simulink model "IEEE_30_Bus_System_with_HVDC"  (R2021a)
settings: Solver=FixedStepDiscrete  StartTime=0.0  StopTime=15  FixedStep=Tss  RelTol=1e-3
InitFcn:
  | Tss=5e-5
  | 
  | Pnom = 20e6
  | Vdc = 40e3
  | 
  | Vbreak_on = Vdc + Vdc*150/800
  | Vbreak_off = Vdc
  | break_status_time = 1.0
  | 
  | Rbrk =  Vdc*Vdc/(1.0*Pnom)
  | 
  | Vg1rms = 33e3*1.0118
  | Lg1 = 20e-6
  | Rg1 = 10e-3
  | f1 = 60.0
  | m_f=27
  | fsw = 10000.0
  | Ilpp = 0.1*Pnom/Vg1rms
  | a = 10.0
  | 
  | ffast = 1.0*fsw
  | Tfast = 1.0/ffast
  | 
  | Rdc = Vdc*Vdc/Pnom
  | 
  | R1 = Vg1rms*Vg1rms / (500*Pnom) / 3.0
  | %L1 = 3.0*1.41*Vg1rms / (2*Vdc) * ((2.0/3.0*Vdc - 1.41*Vg1rms) / (Ilpp*fsw))
  | L1=8e-3
  | %Cf1 = (a+1)/(4*pi*pi*fsw*fsw*Lg1)
  | Cf1=4e-6
  | %C_dc = 100e-10*Pnom
  | C_dc=0.02
  | %R_dump = 1.0/(20.0*pi*f1*Cf1)*10000.0/Pnom
  | R_dump=20
  | 
  | p = -0.135*10.0
  | i = -0.004/2.0
  | 
  | Kp_i = 2*L1*fsw*p / Vdc / 2.0
  | Ki_i = 2*L1*fsw*i / Vdc / 2.0
  | 
  | Tsw = 1/fsw
  | 
  | Vg2rms = 33e3*1.0571
  | Lg2 = 20e-6
  | Rg2 = 10e-3
  | f2 = 60.0
  | fsw2 = 10000.0
  | Il2pp = 0.1*Pnom/Vg2rms
  | a2 = 10.0
  | 
  | R2 = Vg2rms*Vg2rms / (500*Pnom) / 3.0
  | %L2 = 3.0*1.41*Vg2rms / (2*Vdc) * ((2.0/3.0*Vdc - 1.41*Vg2rms) / (Il2pp*fsw2))
  | L2=20e-3
  | %Cf2 = (a2+1)/(4*pi*pi*fsw2*fsw2*Lg2)
  | Cf2=9e-6
  | 
  | %R_dump2 = 1.0/(20.0*pi*f2*Cf2)*10000.0/Pnom
  | R_dump2=20
  | 
  | ... (+10 lines)
undefined symbols (not defined in the file): Angle, DiscIntNeverNeededParam, Magnitude, V_890, Vnom1
libraries: spsThreePhasePISectionLineLib x37, spsThreePhaseVIMeasurementLib x32, spsLoadFlowBusLib x30, spsSeriesRLCBranchLib x27, spsThreePhaseSeriesRLCLoadLib x23, spsVoltageMeasurementLib x17, spsCurrentMeasurementLib x15, spsThreePhaseSourceLib x7, pid_lib x7, spsabctodq0Lib x6, spsFirstOrderFilterLib x4, eeGeneralControl x4
(part 2 of 2)

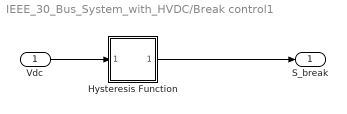
== system IEEE_30_Bus_System_with_HVDC/Break control1 ==
  Vdc : Inport
  Hysteresis Function : Subsystem
  S_break : Outport
  wires:
  Vdc/1 -> Hysteresis Function/1(Input)
  Hysteresis Function/1(Output) -> S_break/1

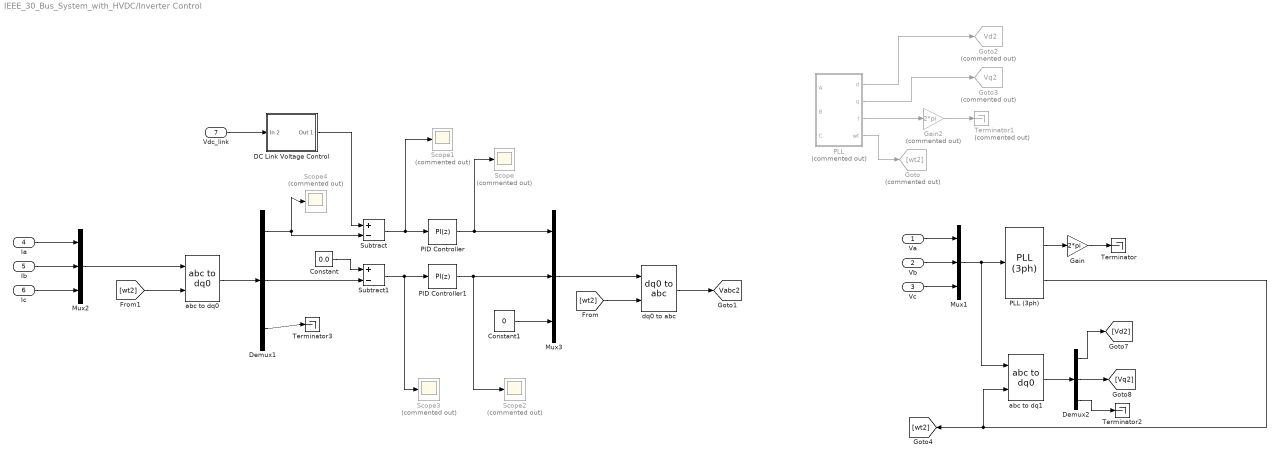
== system IEEE_30_Bus_System_with_HVDC/Inverter Control ==
  Va : Inport
  Vb : Inport  Port=2
  Vc : Inport  Port=3
  Ia : Inport  Port=4
  Ib : Inport  Port=5
  Ic : Inport  Port=6
  Vdc_link : Inport  Port=7
  Constant : Constant  Value=0.0  SampleTime=Tsw2
  Constant1 : Constant  Value=0
  DC Link Voltage Control : Subsystem
  Demux1 : Demux  Outputs=3
  Demux2 : Demux  Outputs=3
  Gain : Gain  Gain=2*pi
  Gain2 : Gain  Commented=on  Gain=2*pi
  Goto : Goto  Commented=on  GotoTag=wt2
  Goto2 : Goto  Commented=on  GotoTag=Vd2  TagVisibility=global
  Goto3 : Goto  Commented=on  GotoTag=Vq2  TagVisibility=global
  Mux1 : Mux  Inputs=3
  Mux2 : Mux  Inputs=3
  Mux3 : Mux  Inputs=3
  PID Controller : pid_lib/PID Controller  Controller=PI  Form=Parallel  TimeDomain=Discrete-time  UseExternalTs=off  SampleTime=-1  IntegratorMethod=Forward Euler  FilterMethod=Forward Euler  ControllerParametersSource=internal  P=Kp_i  I=Ki_i/Tsw2  D=0  UseFilter=on  N=100  TunerSelectOption=Transfer Function Based (PID Tuner App)  InitialConditionSource=internal  InitialConditionForIntegrator=0  InitialConditionForFilter=0  DifferentiatorICPrevScaledInput=0  ExternalReset=none  TrackingMode=off  Kt=1  LimitOutput=on  SatLimitsSource=internal  UpperSaturationLimit=1  LowerSaturationLimit=-1  LinearizeAsGain=on  AntiWindupMode=back-calculation  Kb=Ki_i/Tsw2  POutMin=[]  POutMax=[]  IOutMin=[]  IOutMax=[]  DOutMin=[]  DOutMax=[]  NOutMin=[]  NOutMax=[]  SumOutMin=[]  SumOutMax=[]  SaturationOutMin=[]  SaturationOutMax=[]  PParamMin=[]  PParamMax=[]  IParamMin=[]  IParamMax=[]  DParamMin=[]  DParamMax=[]  NParamMin=[]  NParamMax=[]  KbParamMin=[]  KbParamMax=[]  KtParamMin=[]  KtParamMax=[]  KbOutMin=[]  KbOutMax=[]  KtOutMin=[]  KtOutMax=[]  IntegratorOutMin=[]  IntegratorOutMax=[]  FilterOutMin=[]  FilterOutMax=[]  SumI1OutMin=[]  SumI1OutMax=[]  SumI2OutMin=[]  SumI2OutMax=[]  SumI3OutMin=[]  SumI3OutMax=[]  SumI4OutMin=[]  SumI4OutMax=[]  SumDOutMin=[]  SumDOutMax=[]  DifferentiatorOutMin=[]  DifferentiatorOutMax=[]  FilterDiffOutCoefMin=[]  FilterDiffOutCoefMax=[]  ReciprocalOutMin=[]  ReciprocalOutMax=[]  SumDenOutMin=[]  SumDenOutMax=[]  SumNumOutMin=[]  SumNumOutMax=[]  DivideOutMin=[]  DivideOutMax=[]  UdiffTsProdOutMin=[]  UdiffTsProdOutMax=[]  NTsProdOutMin=[]  NTsProdOutMax=[]  UintegralTsProdOutMin=[]  UintegralTsProdOutMax=[]  UngainTsProdOutMin=[]  UngainTsProdOutMax=[]  IntegratorContinuousStateAttributes=''  IntegratorStateMustResolveToSignalObject=off  IntegratorRTWStateStorageClass=Auto  FilterContinuousStateAttributes=''  FilterStateMustResolveToSignalObject=off  FilterRTWStateStorageClass=Auto  ParallelPVariant=InternalParameters  IdealPVariant=Disabled  IVariant=InternalParameters  DVariant=Disabled  IntegratorVariant=Discrete  SatVariant=Enabled  AWVariant=BackCalculation  PCopyVariant=Disabled  TRVariant=Disabled  FdbkBlocksVariant=Forward  IdealPFdbkVariant=Disabled  SatFdbkVariant=Disabled  DerivativeFilterVariant=Disabled  NVariant=Disabled  NCopyVariant=Disabled_SignalSpec  FilterICVariant=Disabled  IntegratorICVariant=InternalICs  ExternalResetVariant=Disabled  TRSumVariant=Passthrough  SumFdbkVariant=Disabled  SumVariant=Sum_PI  TsampFilterVariant=InternalTs  TsampNgainVariant=Passthrough  TsampIntegralVariant=Passthrough  ExternalSaturationOutDataTypeStr=Inherit: Same as second input
  PID Controller1 : pid_lib/PID Controller  Controller=PI  Form=Parallel  TimeDomain=Discrete-time  UseExternalTs=off  SampleTime=-1  IntegratorMethod=Forward Euler  FilterMethod=Forward Euler  ControllerParametersSource=internal  P=Kp_i  I=Ki_i/Tsw2  D=0  UseFilter=on  N=100  TunerSelectOption=Transfer Function Based (PID Tuner App)  InitialConditionSource=internal  InitialConditionForIntegrator=0  InitialConditionForFilter=0  DifferentiatorICPrevScaledInput=0  ExternalReset=none  TrackingMode=off  Kt=1  LimitOutput=on  SatLimitsSource=internal  UpperSaturationLimit=1  LowerSaturationLimit=-1  LinearizeAsGain=on  AntiWindupMode=back-calculation  Kb=Ki_i/Tsw2  POutMin=[]  POutMax=[]  IOutMin=[]  IOutMax=[]  DOutMin=[]  DOutMax=[]  NOutMin=[]  NOutMax=[]  SumOutMin=[]  SumOutMax=[]  SaturationOutMin=[]  SaturationOutMax=[]  PParamMin=[]  PParamMax=[]  IParamMin=[]  IParamMax=[]  DParamMin=[]  DParamMax=[]  NParamMin=[]  NParamMax=[]  KbParamMin=[]  KbParamMax=[]  KtParamMin=[]  KtParamMax=[]  KbOutMin=[]  KbOutMax=[]  KtOutMin=[]  KtOutMax=[]  IntegratorOutMin=[]  IntegratorOutMax=[]  FilterOutMin=[]  FilterOutMax=[]  SumI1OutMin=[]  SumI1OutMax=[]  SumI2OutMin=[]  SumI2OutMax=[]  SumI3OutMin=[]  SumI3OutMax=[]  SumI4OutMin=[]  SumI4OutMax=[]  SumDOutMin=[]  SumDOutMax=[]  DifferentiatorOutMin=[]  DifferentiatorOutMax=[]  FilterDiffOutCoefMin=[]  FilterDiffOutCoefMax=[]  ReciprocalOutMin=[]  ReciprocalOutMax=[]  SumDenOutMin=[]  SumDenOutMax=[]  SumNumOutMin=[]  SumNumOutMax=[]  DivideOutMin=[]  DivideOutMax=[]  UdiffTsProdOutMin=[]  UdiffTsProdOutMax=[]  NTsProdOutMin=[]  NTsProdOutMax=[]  UintegralTsProdOutMin=[]  UintegralTsProdOutMax=[]  UngainTsProdOutMin=[]  UngainTsProdOutMax=[]  IntegratorContinuousStateAttributes=''  IntegratorStateMustResolveToSignalObject=off  IntegratorRTWStateStorageClass=Auto  FilterContinuousStateAttributes=''  FilterStateMustResolveToSignalObject=off  FilterRTWStateStorageClass=Auto  ParallelPVariant=InternalParameters  IdealPVariant=Disabled  IVariant=InternalParameters  DVariant=Disabled  IntegratorVariant=Discrete  SatVariant=Enabled  AWVariant=BackCalculation  PCopyVariant=Disabled  TRVariant=Disabled  FdbkBlocksVariant=Forward  IdealPFdbkVariant=Disabled  SatFdbkVariant=Disabled  DerivativeFilterVariant=Disabled  NVariant=Disabled  NCopyVariant=Disabled_SignalSpec  FilterICVariant=Disabled  IntegratorICVariant=InternalICs  ExternalResetVariant=Disabled  TRSumVariant=Passthrough  SumFdbkVariant=Disabled  SumVariant=Sum_PI  TsampFilterVariant=InternalTs  TsampNgainVariant=Passthrough  TsampIntegralVariant=Passthrough  ExternalSaturationOutDataTypeStr=Inherit: Same as second input
  PLL : Subsystem  Commented=on
  PLL (3ph) : spsPLL3phLib/PLL (3ph)  Fmin=45  Par_Init=[0, 60]  ParK=[100, 3200, 1]  TcD=1e-4  MaxRateChangeFreq=12  FilterCutOffFreq=25  Ts=Tss  AGC=on
  Scope{,1..4} (5 alike) : Scope  Commented=on
  Subtract : Sum  Inputs=+-
  Subtract1 : Sum  Inputs=+-
  Terminator : Terminator
  Terminator1 : Terminator  Commented=on
  Terminator2 : Terminator
  Terminator3 : Terminator
  abc to dq0 : spsabctodq0Lib/abc to dq0  Alignment=90 degrees behind phase A axis
  abc to dq1 : spsabctodq0Lib/abc to dq0  Alignment=90 degrees behind phase A axis
  dq0 to abc : spsdq0toabcLib/dq0 to abc  Alignment=90 degrees behind phase A axis
  tag scope: Vabc2=global
  wires:
  Ia/1 -> Mux2/1
  Ib/1 -> Mux2/2
  Ic/1 -> Mux2/3
  Mux2/1 -> abc to dq0/1
  abc to dq0/1 -> Demux1/1
  Demux1/2 -> Subtract1/2
  Constant/1 -> Subtract1/1
  Subtract/1 -> Scope1/1, PID Controller/1
  Subtract1/1 -> Scope3/1, PID Controller1/1
  PID Controller/1 -> Scope/1, Mux3/1
  PID Controller1/1 -> Scope2/1, Mux3/2
  Mux3/1 -> dq0 to abc/1
  DC Link Voltage Control/1(Out 1) -> Subtract/1
  PLL/4(wt) -> Goto/1
  PLL/1(d) -> Goto2/1
  PLL/2(q) -> Goto3/1
  Gain2/1 -> Terminator1/1
  PLL/3(f) -> Gain2/1
  Demux2/1 -> [Vd2]
  Gain/1 -> Terminator/1
  Vc/1 -> Mux1/3
  abc to dq1/1 -> Demux2/1
  PLL (3ph)/1 -> Gain/1
  Demux2/2 -> [Vq2]
  Va/1 -> Mux1/1
  Vb/1 -> Mux1/2
  Mux1/1 -> abc to dq1/1, PLL (3ph)/1
  PLL (3ph)/2 -> [wt2], abc to dq1/2
  [wt2] -> dq0 to abc/2
  [wt2] -> abc to dq0/2
  Vdc_link/1 -> DC Link Voltage Control/1(In 2)
  Demux1/1 -> Scope4/1, Subtract/2
  Demux1/3 -> Terminator3/1
  dq0 to abc/1 -> [Vabc2]
  Constant1/1 -> Mux3/3
  Demux2/3 -> Terminator2/1

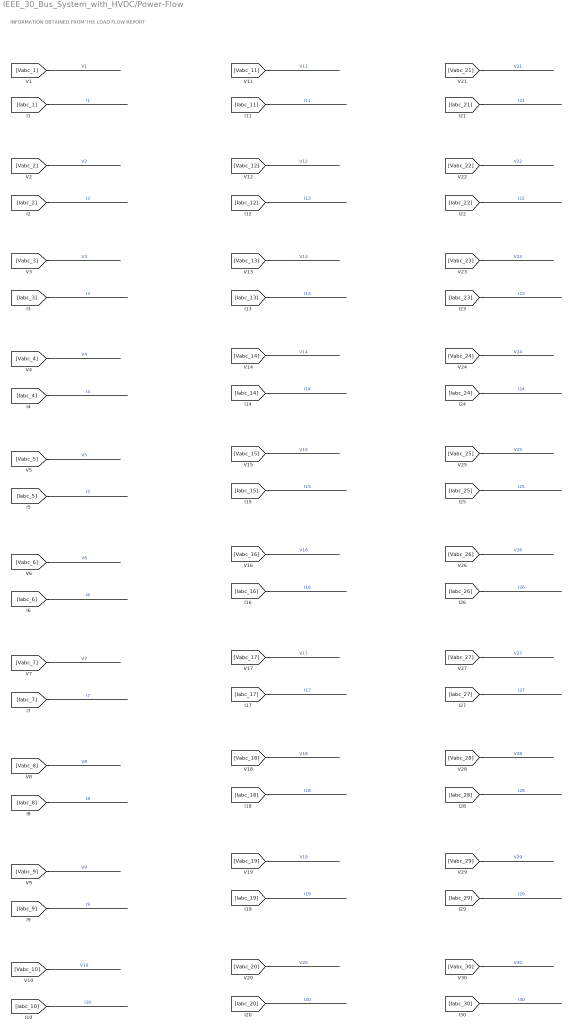
== system IEEE_30_Bus_System_with_HVDC/Power-Flow ==
  note: INFORMATION OBTAINED FROM THE LOAD FLOW REPORT
  wires:
  [Vabc_1] -> ?  "V1"
  [Iabc_1] -> ?  "I1"
  [Vabc_2] -> ?  "V2"
  [Iabc_2] -> ?  "I2"
  [Iabc_3] -> ?  "I3"
  [Vabc_3] -> ?  "V3"
  [Vabc_4] -> ?  "V4"
  [Iabc_4] -> ?  "I4"
  [Vabc_5] -> ?  "V5"
  [Iabc_5] -> ?  "I5"
  [Vabc_6] -> ?  "V6"
  [Iabc_6] -> ?  "I6"
  [Vabc_7] -> ?  "V7"
  [Iabc_7] -> ?  "I7"
  [Vabc_8] -> ?  "V8"
  [Iabc_8] -> ?  "I8"
  [Vabc_9] -> ?  "V9"
  [Iabc_9] -> ?  "I9"
  [Vabc_10] -> ?  "V10"
  [Iabc_10] -> ?  "I10"
  [Iabc_18] -> ?  "I18"
  [Vabc_18] -> ?  "V18"
  [Iabc_13] -> ?  "I13"
  [Vabc_13] -> ?  "V13"
  [Iabc_11] -> ?  "I11"
  [Vabc_16] -> ?  "V16"
  [Iabc_16] -> ?  "I16"
  [Iabc_17] -> ?  "I17"
  [Vabc_17] -> ?  "V17"
  [Vabc_11] -> ?  "V11"
  [Iabc_12] -> ?  "I12"
  [Vabc_20] -> ?  "V20"
  [Iabc_20] -> ?  "I20"
  [Vabc_12] -> ?  "V12"
  [Iabc_19] -> ?  "I19"
  [Iabc_15] -> ?  "I15"
  [Vabc_19] -> ?  "V19"
  [Vabc_15] -> ?  "V15"
  [Vabc_14] -> ?  "V14"
  [Iabc_14] -> ?  "I14"
  [Iabc_26] -> ?  "I26"
  [Vabc_27] -> ?  "V27"
  [Vabc_26] -> ?  "V26"
  [Iabc_21] -> ?  "I21"
  [Vabc_23] -> ?  "V23"
  [Vabc_28] -> ?  "V28"
  [Iabc_27] -> ?  "I27"
  [Iabc_28] -> ?  "I28"
  [Vabc_24] -> ?  "V24"
  [Vabc_25] -> ?  "V25"
  [Iabc_23] -> ?  "I23"
  [Vabc_29] -> ?  "V29"
  [Iabc_24] -> ?  "I24"
  [Iabc_25] -> ?  "I25"
  [Vabc_30] -> ?  "V30"
  [Vabc_22] -> ?  "V22"
  [Iabc_29] -> ?  "I29"
  [Iabc_22] -> ?  "I22"
  [Iabc_30] -> ?  "I30"
  [Vabc_21] -> ?  "V21"

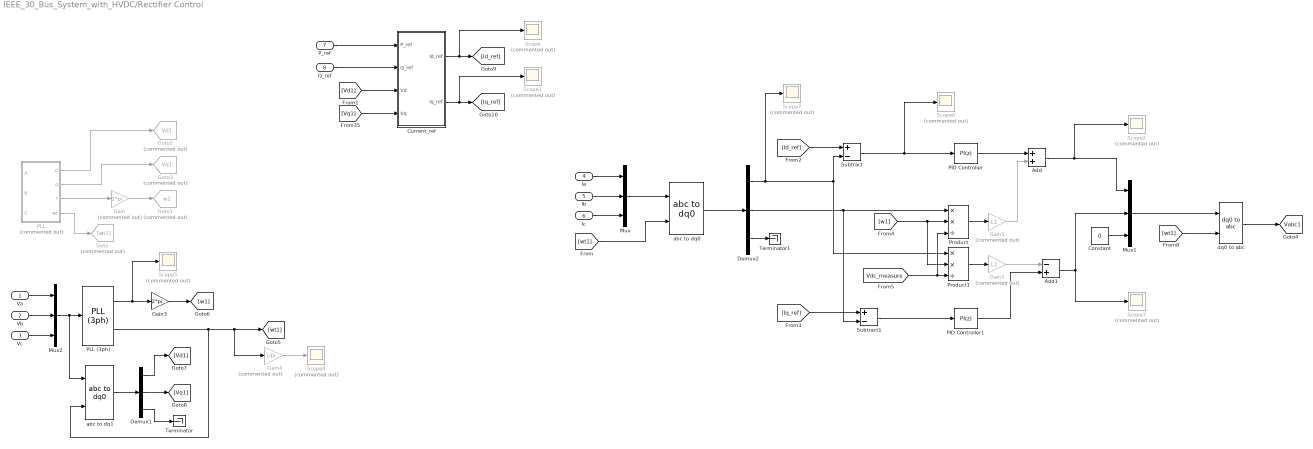
== system IEEE_30_Bus_System_with_HVDC/Rectifier Control ==
  Va : Inport
  Vb : Inport  Port=2
  Vc : Inport  Port=3
  Ia : Inport  Port=4
  Ib : Inport  Port=5
  Ic : Inport  Port=6
  P_ref : Inport  Port=7
  Q_ref : Inport  Port=8
  Add : Sum
  Add1 : Sum  Inputs=-+
  Constant : Constant  Value=0
  Current_ref : Subsystem
  Demux1 : Demux  Outputs=3
  Demux2 : Demux  Outputs=3
  Gain : Gain  Commented=on  Gain=2*pi
  Gain1 : Gain  Commented=on  Gain=L1
  Gain2 : Gain  Commented=on  Gain=L1
  Gain3 : Gain  Gain=2*pi
  Gain4 : Gain  Commented=on  Gain=1/pi
  Goto : Goto  Commented=on  GotoTag=wt1
  Goto1 : Goto  Commented=on  GotoTag=w1  TagVisibility=global
  Goto2 : Goto  Commented=on  GotoTag=Vd1  TagVisibility=global
  Goto3 : Goto  Commented=on  GotoTag=Vq1  TagVisibility=global
  Mux : Mux  Inputs=3
  Mux1 : Mux  Inputs=3
  Mux2 : Mux  Inputs=3
  PID Controller : pid_lib/PID Controller  Controller=PI  Form=Parallel  TimeDomain=Discrete-time  UseExternalTs=off  SampleTime=-1  IntegratorMethod=Forward Euler  FilterMethod=Forward Euler  ControllerParametersSource=internal  P=Kp_i  I=Ki_i/Tsw  D=0  UseFilter=on  N=100  TunerSelectOption=Transfer Function Based (PID Tuner App)  InitialConditionSource=internal  InitialConditionForIntegrator=0  InitialConditionForFilter=0  DifferentiatorICPrevScaledInput=0  ExternalReset=none  TrackingMode=off  Kt=1  LimitOutput=on  SatLimitsSource=internal  UpperSaturationLimit=1  LowerSaturationLimit=-1  LinearizeAsGain=on  AntiWindupMode=back-calculation  Kb=Ki_i/Tsw  POutMin=[]  POutMax=[]  IOutMin=[]  IOutMax=[]  DOutMin=[]  DOutMax=[]  NOutMin=[]  NOutMax=[]  SumOutMin=[]  SumOutMax=[]  SaturationOutMin=[]  SaturationOutMax=[]  PParamMin=[]  PParamMax=[]  IParamMin=[]  IParamMax=[]  DParamMin=[]  DParamMax=[]  NParamMin=[]  NParamMax=[]  KbParamMin=[]  KbParamMax=[]  KtParamMin=[]  KtParamMax=[]  KbOutMin=[]  KbOutMax=[]  KtOutMin=[]  KtOutMax=[]  IntegratorOutMin=[]  IntegratorOutMax=[]  FilterOutMin=[]  FilterOutMax=[]  SumI1OutMin=[]  SumI1OutMax=[]  SumI2OutMin=[]  SumI2OutMax=[]  SumI3OutMin=[]  SumI3OutMax=[]  SumI4OutMin=[]  SumI4OutMax=[]  SumDOutMin=[]  SumDOutMax=[]  DifferentiatorOutMin=[]  DifferentiatorOutMax=[]  FilterDiffOutCoefMin=[]  FilterDiffOutCoefMax=[]  ReciprocalOutMin=[]  ReciprocalOutMax=[]  SumDenOutMin=[]  SumDenOutMax=[]  SumNumOutMin=[]  SumNumOutMax=[]  DivideOutMin=[]  DivideOutMax=[]  UdiffTsProdOutMin=[]  UdiffTsProdOutMax=[]  NTsProdOutMin=[]  NTsProdOutMax=[]  UintegralTsProdOutMin=[]  UintegralTsProdOutMax=[]  UngainTsProdOutMin=[]  UngainTsProdOutMax=[]  IntegratorContinuousStateAttributes=''  IntegratorStateMustResolveToSignalObject=off  IntegratorRTWStateStorageClass=Auto  FilterContinuousStateAttributes=''  FilterStateMustResolveToSignalObject=off  FilterRTWStateStorageClass=Auto  ParallelPVariant=InternalParameters  IdealPVariant=Disabled  IVariant=InternalParameters  DVariant=Disabled  IntegratorVariant=Discrete  SatVariant=Enabled  AWVariant=BackCalculation  PCopyVariant=Disabled  TRVariant=Disabled  FdbkBlocksVariant=Forward  IdealPFdbkVariant=Disabled  SatFdbkVariant=Disabled  DerivativeFilterVariant=Disabled  NVariant=Disabled  NCopyVariant=Disabled_SignalSpec  FilterICVariant=Disabled  IntegratorICVariant=InternalICs  ExternalResetVariant=Disabled  TRSumVariant=Passthrough  SumFdbkVariant=Disabled  SumVariant=Sum_PI  TsampFilterVariant=InternalTs  TsampNgainVariant=Passthrough  TsampIntegralVariant=Passthrough  ExternalSaturationOutDataTypeStr=Inherit: Same as second input
  PID Controller1 : pid_lib/PID Controller  Controller=PI  Form=Parallel  TimeDomain=Discrete-time  UseExternalTs=off  SampleTime=-1  IntegratorMethod=Forward Euler  FilterMethod=Forward Euler  ControllerParametersSource=internal  P=Kp_i  I=Ki_i/Tsw  D=0  UseFilter=on  N=100  TunerSelectOption=Transfer Function Based (PID Tuner App)  InitialConditionSource=internal  InitialConditionForIntegrator=0  InitialConditionForFilter=0  DifferentiatorICPrevScaledInput=0  ExternalReset=none  TrackingMode=off  Kt=1  LimitOutput=on  SatLimitsSource=internal  UpperSaturationLimit=1  LowerSaturationLimit=-1  LinearizeAsGain=on  AntiWindupMode=back-calculation  Kb=Ki_i/Tsw  POutMin=[]  POutMax=[]  IOutMin=[]  IOutMax=[]  DOutMin=[]  DOutMax=[]  NOutMin=[]  NOutMax=[]  SumOutMin=[]  SumOutMax=[]  SaturationOutMin=[]  SaturationOutMax=[]  PParamMin=[]  PParamMax=[]  IParamMin=[]  IParamMax=[]  DParamMin=[]  DParamMax=[]  NParamMin=[]  NParamMax=[]  KbParamMin=[]  KbParamMax=[]  KtParamMin=[]  KtParamMax=[]  KbOutMin=[]  KbOutMax=[]  KtOutMin=[]  KtOutMax=[]  IntegratorOutMin=[]  IntegratorOutMax=[]  FilterOutMin=[]  FilterOutMax=[]  SumI1OutMin=[]  SumI1OutMax=[]  SumI2OutMin=[]  SumI2OutMax=[]  SumI3OutMin=[]  SumI3OutMax=[]  SumI4OutMin=[]  SumI4OutMax=[]  SumDOutMin=[]  SumDOutMax=[]  DifferentiatorOutMin=[]  DifferentiatorOutMax=[]  FilterDiffOutCoefMin=[]  FilterDiffOutCoefMax=[]  ReciprocalOutMin=[]  ReciprocalOutMax=[]  SumDenOutMin=[]  SumDenOutMax=[]  SumNumOutMin=[]  SumNumOutMax=[]  DivideOutMin=[]  DivideOutMax=[]  UdiffTsProdOutMin=[]  UdiffTsProdOutMax=[]  NTsProdOutMin=[]  NTsProdOutMax=[]  UintegralTsProdOutMin=[]  UintegralTsProdOutMax=[]  UngainTsProdOutMin=[]  UngainTsProdOutMax=[]  IntegratorContinuousStateAttributes=''  IntegratorStateMustResolveToSignalObject=off  IntegratorRTWStateStorageClass=Auto  FilterContinuousStateAttributes=''  FilterStateMustResolveToSignalObject=off  FilterRTWStateStorageClass=Auto  ParallelPVariant=InternalParameters  IdealPVariant=Disabled  IVariant=InternalParameters  DVariant=Disabled  IntegratorVariant=Discrete  SatVariant=Enabled  AWVariant=BackCalculation  PCopyVariant=Disabled  TRVariant=Disabled  FdbkBlocksVariant=Forward  IdealPFdbkVariant=Disabled  SatFdbkVariant=Disabled  DerivativeFilterVariant=Disabled  NVariant=Disabled  NCopyVariant=Disabled_SignalSpec  FilterICVariant=Disabled  IntegratorICVariant=InternalICs  ExternalResetVariant=Disabled  TRSumVariant=Passthrough  SumFdbkVariant=Disabled  SumVariant=Sum_PI  TsampFilterVariant=InternalTs  TsampNgainVariant=Passthrough  TsampIntegralVariant=Passthrough  ExternalSaturationOutDataTypeStr=Inherit: Same as second input
  PLL : Subsystem  Commented=on
  PLL (3ph) : spsPLL3phLib/PLL (3ph)  Fmin=45  Par_Init=[0, 60]  ParK=[100, 3200, 1]  TcD=1e-4  MaxRateChangeFreq=12  FilterCutOffFreq=25  Ts=Tss  AGC=on
  Product : Product  Inputs=**/
  Product1 : Product  Inputs=**/
  Scope{,1..7} (8 alike) : Scope  Commented=on
  Subtract : Sum  Inputs=+-
  Subtract1 : Sum  Inputs=+-
  Terminator : Terminator
  Terminator1 : Terminator
  abc to dq0 : spsabctodq0Lib/abc to dq0  Alignment=90 degrees behind phase A axis
  abc to dq1 : spsabctodq0Lib/abc to dq0  Alignment=90 degrees behind phase A axis
  dq0 to abc : spsdq0toabcLib/dq0 to abc  Alignment=90 degrees behind phase A axis
  tag scope: Vabc1=global
  wires:
  PLL/4(wt) -> Goto/1
  PLL/3(f) -> Gain/1
  Gain/1 -> Goto1/1
  PLL/1(d) -> Goto2/1
  PLL/2(q) -> Goto3/1
  [wt1] -> abc to dq0/2
  abc to dq0/1 -> Demux2/1
  Demux2/3 -> Terminator1/1
  Mux/1 -> abc to dq0/1
  Demux2/1 -> Scope7/1, Product1/1, Subtract/2
  Demux2/2 -> Subtract1/2, Product/1
  [w1] -> Product1/2, Product/2
  [Vdc_measure] -> Product/3, Product1/3
  [wt1] -> dq0 to abc/2
  Subtract/1 -> Scope6/1, PID Controller/1
  Subtract1/1 -> PID Controller1/1
  PID Controller1/1 -> Add1/2
  Product/1 -> Gain1/1
  Product1/1 -> Gain2/1
  Gain2/1 -> Add1/1
  dq0 to abc/1 -> [Vabc1]
  Ia/1 -> Mux/1
  Ic/1 -> Mux/3
  Ib/1 -> Mux/2
  Add/1 -> Mux1/1, Scope2/1
  PID Controller/1 -> Add/1
  Gain1/1 -> Add/2
  Demux1/2 -> [Vq1]
  abc to dq1/1 -> Demux1/1
  Mux2/1 -> abc to dq1/1, PLL (3ph)/1
  PLL (3ph)/1 -> Scope5/1, Gain3/1
  Gain3/1 -> [w1]
  Demux1/1 -> [Vd1]
  PLL (3ph)/2 -> abc to dq1/2, Gain4/1, [wt1]
  [Vq1] -> Current_ref/4(Vq)
  [Vd1] -> Current_ref/3(Vd)
  Mux1/1 -> dq0 to abc/1
  Add1/1 -> Mux1/2, Scope3/1
  Constant/1 -> Mux1/3
  P_ref/1 -> Current_ref/1(P_ref)
  Demux1/3 -> Terminator/1
  Va/1 -> Mux2/1
  Vb/1 -> Mux2/2
  Vc/1 -> Mux2/3
  Q_ref/1 -> Current_ref/2(Q_ref)
  Current_ref/1(Id_ref) -> Scope/1, [Id_ref]
  Current_ref/2(Iq_ref) -> Scope1/1, [Iq_ref]
  [Id_ref] -> Subtract/1
  [Iq_ref] -> Subtract1/1
  Gain4/1 -> Scope4/1

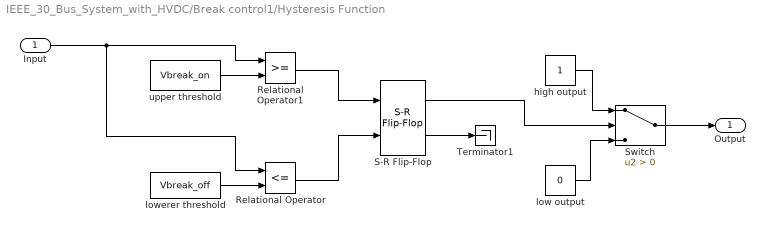
== system IEEE_30_Bus_System_with_HVDC/Break control1/Hysteresis Function ==
  Input : Inport
  Relational Operator : RelationalOperator  Operator=<=  OutDataTypeStr=boolean  RndMeth=Simplest
  Relational Operator1 : RelationalOperator  OutDataTypeStr=boolean  RndMeth=Simplest
  S-R Flip-Flop : simulink_extras/Flip Flops/S-R Flip-Flop  initial_condition=0
  Switch : Switch  Criteria=u2 > Threshold
  Terminator1 : Terminator
  high output : Constant  SampleTime=Tfast
  low output : Constant  Value=0  SampleTime=Tfast
  lowerer threshold : Constant  Value=Vbreak_off  SampleTime=Tfast
  upper threshold : Constant  Value=Vbreak_on  SampleTime=Tfast
  Output : Outport
  wires:
  lowerer threshold/1 -> Relational Operator/2
  upper threshold/1 -> Relational Operator1/2
  Relational Operator1/1 -> S-R Flip-Flop/1
  Relational Operator/1 -> S-R Flip-Flop/2
  S-R Flip-Flop/2 -> Terminator1/1
  S-R Flip-Flop/1 -> Switch/2
  high output/1 -> Switch/1
  low output/1 -> Switch/3
  Input/1 -> Relational Operator1/1, Relational Operator/1
  Switch/1 -> Output/1

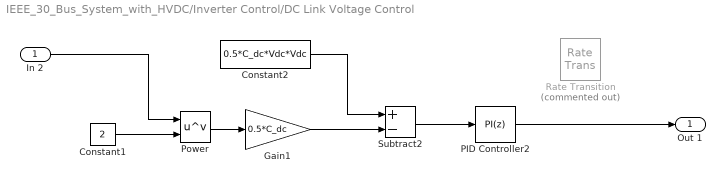
== system IEEE_30_Bus_System_with_HVDC/Inverter Control/DC Link Voltage Control ==
  In 2 : Inport
  Constant1 : Constant  Value=2  SampleTime=Tslow
  Constant2 : Constant  Value=0.5*C_dc*Vdc*Vdc  SampleTime=Tslow
  Gain1 : Gain  Gain=0.5*C_dc
  PID Controller2 : pid_lib/PID Controller  Controller=PI  Form=Parallel  TimeDomain=Discrete-time  UseExternalTs=off  SampleTime=-1  IntegratorMethod=Forward Euler  FilterMethod=Forward Euler  ControllerParametersSource=internal  P=Kp_v  I=Ki_v/Tslow  D=0  UseFilter=on  N=100  TunerSelectOption=Transfer Function Based (PID Tuner App)  InitialConditionSource=internal  InitialConditionForIntegrator=0  InitialConditionForFilter=0  DifferentiatorICPrevScaledInput=0  ExternalReset=none  TrackingMode=off  Kt=1  LimitOutput=on  SatLimitsSource=internal  UpperSaturationLimit=Imax  LowerSaturationLimit=-Imax  LinearizeAsGain=on  AntiWindupMode=back-calculation  Kb=Ki_v/Tslow  POutMin=[]  POutMax=[]  IOutMin=[]  IOutMax=[]  DOutMin=[]  DOutMax=[]  NOutMin=[]  NOutMax=[]  SumOutMin=[]  SumOutMax=[]  SaturationOutMin=[]  SaturationOutMax=[]  PParamMin=[]  PParamMax=[]  IParamMin=[]  IParamMax=[]  DParamMin=[]  DParamMax=[]  NParamMin=[]  NParamMax=[]  KbParamMin=[]  KbParamMax=[]  KtParamMin=[]  KtParamMax=[]  KbOutMin=[]  KbOutMax=[]  KtOutMin=[]  KtOutMax=[]  IntegratorOutMin=[]  IntegratorOutMax=[]  FilterOutMin=[]  FilterOutMax=[]  SumI1OutMin=[]  SumI1OutMax=[]  SumI2OutMin=[]  SumI2OutMax=[]  SumI3OutMin=[]  SumI3OutMax=[]  SumI4OutMin=[]  SumI4OutMax=[]  SumDOutMin=[]  SumDOutMax=[]  DifferentiatorOutMin=[]  DifferentiatorOutMax=[]  FilterDiffOutCoefMin=[]  FilterDiffOutCoefMax=[]  ReciprocalOutMin=[]  ReciprocalOutMax=[]  SumDenOutMin=[]  SumDenOutMax=[]  SumNumOutMin=[]  SumNumOutMax=[]  DivideOutMin=[]  DivideOutMax=[]  UdiffTsProdOutMin=[]  UdiffTsProdOutMax=[]  NTsProdOutMin=[]  NTsProdOutMax=[]  UintegralTsProdOutMin=[]  UintegralTsProdOutMax=[]  UngainTsProdOutMin=[]  UngainTsProdOutMax=[]  IntegratorContinuousStateAttributes=''  IntegratorStateMustResolveToSignalObject=off  IntegratorRTWStateStorageClass=Auto  FilterContinuousStateAttributes=''  FilterStateMustResolveToSignalObject=off  FilterRTWStateStorageClass=Auto  ParallelPVariant=InternalParameters  IdealPVariant=Disabled  IVariant=InternalParameters  DVariant=Disabled  IntegratorVariant=Discrete  SatVariant=Enabled  AWVariant=BackCalculation  PCopyVariant=Disabled  TRVariant=Disabled  FdbkBlocksVariant=Forward  IdealPFdbkVariant=Disabled  SatFdbkVariant=Disabled  DerivativeFilterVariant=Disabled  NVariant=Disabled  NCopyVariant=Disabled_SignalSpec  FilterICVariant=Disabled  IntegratorICVariant=InternalICs  ExternalResetVariant=Disabled  TRSumVariant=Passthrough  SumFdbkVariant=Disabled  SumVariant=Sum_PI  TsampFilterVariant=InternalTs  TsampNgainVariant=Passthrough  TsampIntegralVariant=Passthrough  ExternalSaturationOutDataTypeStr=Inherit: Same as second input
  Power : Math  Operator=pow  SaturateOnIntegerOverflow=on
  Rate Transition : RateTransition  Commented=on  OutPortSampleTime=Tsw2
  Subtract2 : Sum  Inputs=+-
  Out 1 : Outport
  wires:
  Subtract2/1 -> PID Controller2/1
  Power/1 -> Gain1/1
  Gain1/1 -> Subtract2/2
  In 2/1 -> Power/1
  Constant1/1 -> Power/2
  Constant2/1 -> Subtract2/1
  PID Controller2/1 -> Out 1/1

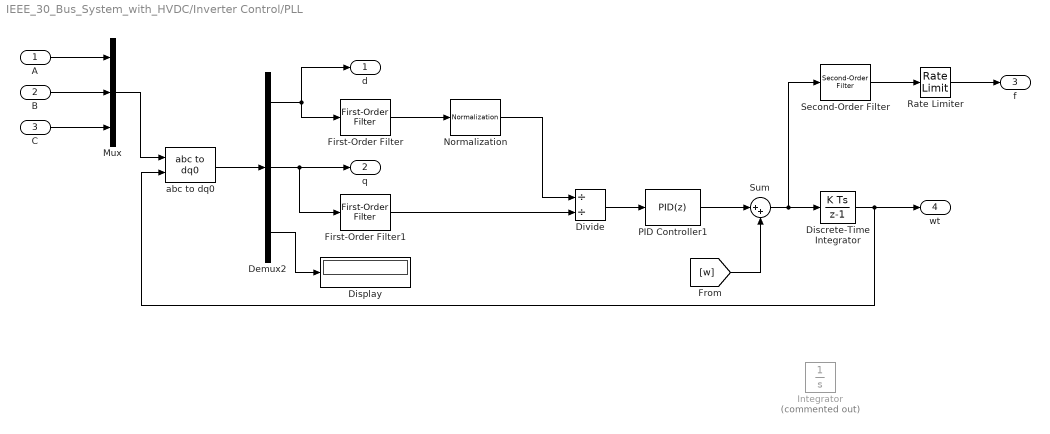
== system IEEE_30_Bus_System_with_HVDC/Inverter Control/PLL ==
  A : Inport
  B : Inport  Port=2
  C : Inport  Port=3
  Demux2 : Demux  Outputs=3
  Discrete-Time Integrator : DiscreteIntegrator  SampleTime=-1  ICPrevOutput=DiscIntNeverNeededParam  ICPrevScaledInput=DiscIntNeverNeededParam
  Display : Display
  Divide : Product  Inputs=//
  First-Order Filter : spsFirstOrderFilterLib/First-Order Filter  FilterType=Lowpass  Tc=10e-3  Ts=Tss  Initialize=on  Vac_Init=[0, 0, 60]  Vdc_Init=0  PlotResponse=off  FreqRange="[0,  200,  1]"
  First-Order Filter1 : spsFirstOrderFilterLib/First-Order Filter  FilterType=Lowpass  Tc=10e-3  Ts=Tss  Initialize=on  Vac_Init=[0, 0, 60]  Vdc_Init=0  PlotResponse=off  FreqRange="[0,  200,  1]"
  Integrator : Integrator  Commented=on
  Mux : Mux  Inputs=3
  Normalization : dspmathops/Normalization  NormType=2-norm  Bias=1e-10  NormOver=Each column  Dimension=1  roundingMode=Floor  overflowMode=off  accumDataTypeStr=Inherit: Same as product output  accumLastDataTypeStr=Inherit: Same as product output  outputDataTypeStr=Inherit: Same as product output  outputMin=[]  outputMax=[]  outputLastDataTypeStr=Inherit: Same as product output
  PID Controller1 : pid_lib/PID Controller  Controller=PID  Form=Parallel  TimeDomain=Discrete-time  UseExternalTs=off  SampleTime=-1  IntegratorMethod=Forward Euler  FilterMethod=Forward Euler  ControllerParametersSource=internal  P=100  I=3200  D=1  UseFilter=on  N=100  TunerSelectOption=Transfer Function Based (PID Tuner App)  InitialConditionSource=internal  InitialConditionForIntegrator=0  InitialConditionForFilter=0  DifferentiatorICPrevScaledInput=0  ExternalReset=none  TrackingMode=off  Kt=1  LimitOutput=on  SatLimitsSource=internal  UpperSaturationLimit=1e4  LowerSaturationLimit=-1e4  LinearizeAsGain=on  AntiWindupMode=back-calculation  Kb=1  POutMin=[]  POutMax=[]  IOutMin=[]  IOutMax=[]  DOutMin=[]  DOutMax=[]  NOutMin=[]  NOutMax=[]  SumOutMin=[]  SumOutMax=[]  SaturationOutMin=[]  SaturationOutMax=[]  PParamMin=[]  PParamMax=[]  IParamMin=[]  IParamMax=[]  DParamMin=[]  DParamMax=[]  NParamMin=[]  NParamMax=[]  KbParamMin=[]  KbParamMax=[]  KtParamMin=[]  KtParamMax=[]  KbOutMin=[]  KbOutMax=[]  KtOutMin=[]  KtOutMax=[]  IntegratorOutMin=[]  IntegratorOutMax=[]  FilterOutMin=[]  FilterOutMax=[]  SumI1OutMin=[]  SumI1OutMax=[]  SumI2OutMin=[]  SumI2OutMax=[]  SumI3OutMin=[]  SumI3OutMax=[]  SumI4OutMin=[]  SumI4OutMax=[]  SumDOutMin=[]  SumDOutMax=[]  DifferentiatorOutMin=[]  DifferentiatorOutMax=[]  FilterDiffOutCoefMin=[]  FilterDiffOutCoefMax=[]  ReciprocalOutMin=[]  ReciprocalOutMax=[]  SumDenOutMin=[]  SumDenOutMax=[]  SumNumOutMin=[]  SumNumOutMax=[]  DivideOutMin=[]  DivideOutMax=[]  UdiffTsProdOutMin=[]  UdiffTsProdOutMax=[]  NTsProdOutMin=[]  NTsProdOutMax=[]  UintegralTsProdOutMin=[]  UintegralTsProdOutMax=[]  UngainTsProdOutMin=[]  UngainTsProdOutMax=[]  IntegratorContinuousStateAttributes=''  IntegratorStateMustResolveToSignalObject=off  IntegratorRTWStateStorageClass=Auto  FilterContinuousStateAttributes=''  FilterStateMustResolveToSignalObject=off  FilterRTWStateStorageClass=Auto  ParallelPVariant=InternalParameters  IdealPVariant=Disabled  IVariant=InternalParameters  DVariant=InternalParameters  IntegratorVariant=Discrete  SatVariant=Enabled  AWVariant=BackCalculation  PCopyVariant=Disabled  TRVariant=Disabled  FdbkBlocksVariant=Forward  IdealPFdbkVariant=Disabled  SatFdbkVariant=Disabled  DerivativeFilterVariant=ForwardEulerFilter  NVariant=InternalParameters  NCopyVariant=Disabled  FilterICVariant=InternalICsFilter  IntegratorICVariant=InternalICs  ExternalResetVariant=Disabled  TRSumVariant=Passthrough  SumFdbkVariant=Disabled  SumVariant=Sum_PID  TsampFilterVariant=InternalTs  TsampNgainVariant=Passthrough  TsampIntegralVariant=Passthrough  ExternalSaturationOutDataTypeStr=Inherit: Same as second input
  Rate Limiter : RateLimiter  SampleTimeMode=inherited
  Second-Order Filter : spsSecondOrderFilterLib/Second-Order Filter  FilterType=Lowpass  Fo=120  Zeta=0.707  Ts=Tss  Initialize=on  Vac_Init="[0,  0,  60]"  Vdc_Init=0  PlotResponse=off  FreqRange=[0, 500, 1]
      settings: SourceProductBaseCode=PS
  Sum : Sum  Inputs=|++
  abc to dq0 : spsabctodq0Lib/abc to dq0  Alignment=90 degrees behind phase A axis
  d : Outport
  q : Outport  Port=2
  f : Outport  Port=3
  wt : Outport  Port=4
  wires:
  A/1 -> Mux/1
  B/1 -> Mux/2
  C/1 -> Mux/3
  Mux/1 -> abc to dq0/1
  abc to dq0/1 -> Demux2/1
  Demux2/1 -> First-Order Filter/1, d/1
  Demux2/2 -> First-Order Filter1/1, q/1
  First-Order Filter1/1 -> Divide/2
  Divide/1 -> PID Controller1/1
  PID Controller1/1 -> Sum/1
  Second-Order Filter/1 -> Rate Limiter/1
  Normalization/1 -> Divide/1
  First-Order Filter/1 -> Normalization/1
  Sum/1 -> Discrete-Time Integrator/1, Second-Order Filter/1
  Discrete-Time Integrator/1 -> wt/1, abc to dq0/2
  Rate Limiter/1 -> f/1
  [w] -> Sum/2
  Demux2/3 -> Display/1

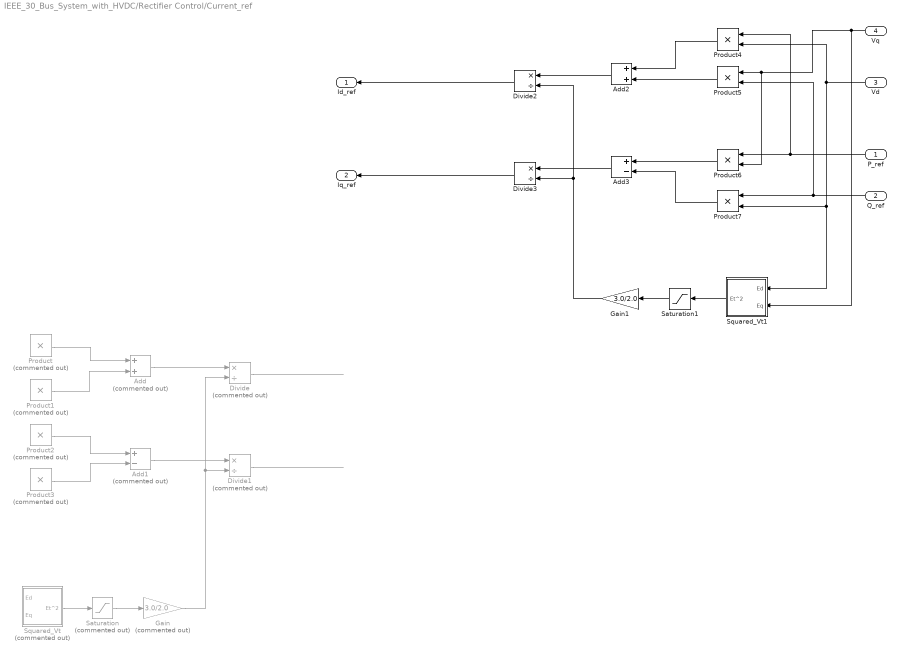
== system IEEE_30_Bus_System_with_HVDC/Rectifier Control/Current_ref ==
  P_ref : Inport
  Q_ref : Inport  Port=2
  Vd : Inport  Port=3
  Vq : Inport  Port=4
  Add : Sum  Commented=on
  Add1 : Sum  Commented=on  Inputs=+-
  Add2 : Sum
  Add3 : Sum  Inputs=+-
  Divide : Product  Commented=on  Inputs=*/
  Divide1 : Product  Commented=on  Inputs=*/
  Divide2 : Product  Inputs=*/
  Divide3 : Product  Inputs=*/
  Gain : Gain  Commented=on  Gain=3.0/2.0
  Gain1 : Gain  Gain=3.0/2.0
  Product{,1..3} (4 alike) : Product  Commented=on
  Product{4..7} (4 alike) : Product
  Saturation : Saturate  Commented=on  UpperLimit=inf  LowerLimit=0.1
  Saturation1 : Saturate  UpperLimit=inf  LowerLimit=0.1
  Squared_Vt : Subsystem  Commented=on
  Squared_Vt1 : Subsystem
  Id_ref : Outport
  Iq_ref : Outport  Port=2
  wires:
  Add2/1 -> Divide2/1
  Add3/1 -> Divide3/1
  Product5/1 -> Add2/2
  Product6/1 -> Add3/1
  Product4/1 -> Add2/1
  Product7/1 -> Add3/2
  Squared_Vt1/1(Et^2) -> Saturation1/1
  Saturation1/1 -> Gain1/1
  Gain1/1 -> Divide2/2, Divide3/2
  Gain/1 -> Divide1/2, Divide/2
  Product/1 -> Add/1
  Add1/1 -> Divide1/1
  Add/1 -> Divide/1
  Saturation/1 -> Gain/1
  Product2/1 -> Add1/1
  Divide1/1 -> ?
  Squared_Vt/1(Et^2) -> Saturation/1
  ? -> Product3/1, Squared_Vt/1(Ed), Product/1
  ? -> Product3/2, Product1/1
  Product1/1 -> Add/2
  ? -> Product2/1, Product/2
  ? -> Squared_Vt/2(Eq), Product2/2, Product1/2
  Product3/1 -> Add1/2
  Divide/1 -> ?
  Divide2/1 -> Id_ref/1
  Divide3/1 -> Iq_ref/1
  Vq/1 -> Squared_Vt1/2(Eq), Product6/2, Product5/1
  Vd/1 -> Squared_Vt1/1(Ed), Product7/2, Product4/2
  P_ref/1 -> Product6/1, Product4/1
  Q_ref/1 -> Product5/2, Product7/1

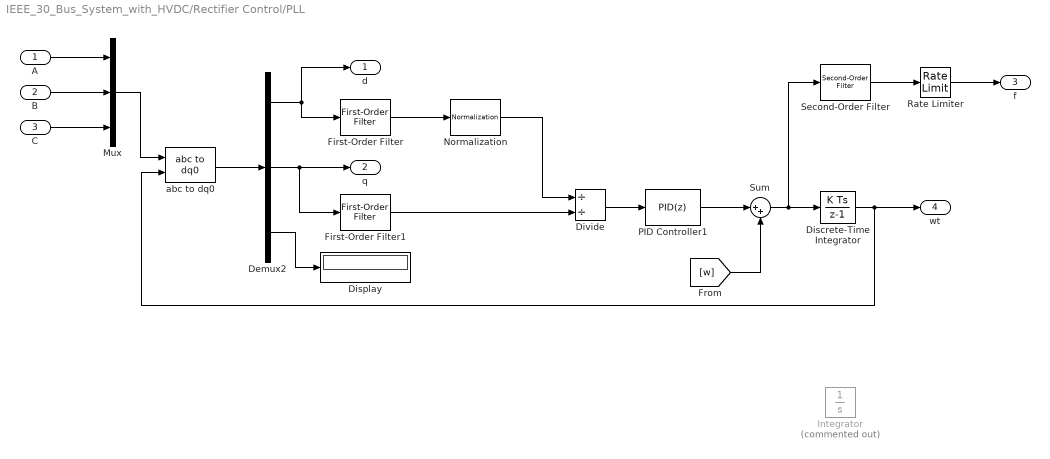
== system IEEE_30_Bus_System_with_HVDC/Rectifier Control/PLL ==
  A : Inport
  B : Inport  Port=2
  C : Inport  Port=3
  Demux2 : Demux  Outputs=3
  Discrete-Time Integrator : DiscreteIntegrator  SampleTime=-1  ICPrevOutput=DiscIntNeverNeededParam  ICPrevScaledInput=DiscIntNeverNeededParam
  Display : Display
  Divide : Product  Inputs=//
  First-Order Filter : spsFirstOrderFilterLib/First-Order Filter  FilterType=Lowpass  Tc=10e-3  Ts=Tss  Initialize=on  Vac_Init=[0, 0, 60]  Vdc_Init=0  PlotResponse=off  FreqRange="[0,  200,  1]"
  First-Order Filter1 : spsFirstOrderFilterLib/First-Order Filter  FilterType=Lowpass  Tc=10e-3  Ts=Tss  Initialize=on  Vac_Init=[0, 0, 60]  Vdc_Init=0  PlotResponse=off  FreqRange="[0,  200,  1]"
  Integrator : Integrator  Commented=on
  Mux : Mux  Inputs=3
  Normalization : dspmathops/Normalization  NormType=2-norm  Bias=1e-10  NormOver=Each column  Dimension=1  roundingMode=Floor  overflowMode=off  accumDataTypeStr=Inherit: Same as product output  accumLastDataTypeStr=Inherit: Same as product output  outputDataTypeStr=Inherit: Same as product output  outputMin=[]  outputMax=[]  outputLastDataTypeStr=Inherit: Same as product output
  PID Controller1 : pid_lib/PID Controller  Controller=PID  Form=Parallel  TimeDomain=Discrete-time  UseExternalTs=off  SampleTime=-1  IntegratorMethod=Forward Euler  FilterMethod=Forward Euler  ControllerParametersSource=internal  P=100  I=3200  D=1  UseFilter=on  N=100  TunerSelectOption=Transfer Function Based (PID Tuner App)  InitialConditionSource=internal  InitialConditionForIntegrator=0  InitialConditionForFilter=0  DifferentiatorICPrevScaledInput=0  ExternalReset=none  TrackingMode=off  Kt=1  LimitOutput=on  SatLimitsSource=internal  UpperSaturationLimit=1e4  LowerSaturationLimit=-1e4  LinearizeAsGain=on  AntiWindupMode=back-calculation  Kb=1  POutMin=[]  POutMax=[]  IOutMin=[]  IOutMax=[]  DOutMin=[]  DOutMax=[]  NOutMin=[]  NOutMax=[]  SumOutMin=[]  SumOutMax=[]  SaturationOutMin=[]  SaturationOutMax=[]  PParamMin=[]  PParamMax=[]  IParamMin=[]  IParamMax=[]  DParamMin=[]  DParamMax=[]  NParamMin=[]  NParamMax=[]  KbParamMin=[]  KbParamMax=[]  KtParamMin=[]  KtParamMax=[]  KbOutMin=[]  KbOutMax=[]  KtOutMin=[]  KtOutMax=[]  IntegratorOutMin=[]  IntegratorOutMax=[]  FilterOutMin=[]  FilterOutMax=[]  SumI1OutMin=[]  SumI1OutMax=[]  SumI2OutMin=[]  SumI2OutMax=[]  SumI3OutMin=[]  SumI3OutMax=[]  SumI4OutMin=[]  SumI4OutMax=[]  SumDOutMin=[]  SumDOutMax=[]  DifferentiatorOutMin=[]  DifferentiatorOutMax=[]  FilterDiffOutCoefMin=[]  FilterDiffOutCoefMax=[]  ReciprocalOutMin=[]  ReciprocalOutMax=[]  SumDenOutMin=[]  SumDenOutMax=[]  SumNumOutMin=[]  SumNumOutMax=[]  DivideOutMin=[]  DivideOutMax=[]  UdiffTsProdOutMin=[]  UdiffTsProdOutMax=[]  NTsProdOutMin=[]  NTsProdOutMax=[]  UintegralTsProdOutMin=[]  UintegralTsProdOutMax=[]  UngainTsProdOutMin=[]  UngainTsProdOutMax=[]  IntegratorContinuousStateAttributes=''  IntegratorStateMustResolveToSignalObject=off  IntegratorRTWStateStorageClass=Auto  FilterContinuousStateAttributes=''  FilterStateMustResolveToSignalObject=off  FilterRTWStateStorageClass=Auto  ParallelPVariant=InternalParameters  IdealPVariant=Disabled  IVariant=InternalParameters  DVariant=InternalParameters  IntegratorVariant=Discrete  SatVariant=Enabled  AWVariant=BackCalculation  PCopyVariant=Disabled  TRVariant=Disabled  FdbkBlocksVariant=Forward  IdealPFdbkVariant=Disabled  SatFdbkVariant=Disabled  DerivativeFilterVariant=ForwardEulerFilter  NVariant=InternalParameters  NCopyVariant=Disabled  FilterICVariant=InternalICsFilter  IntegratorICVariant=InternalICs  ExternalResetVariant=Disabled  TRSumVariant=Passthrough  SumFdbkVariant=Disabled  SumVariant=Sum_PID  TsampFilterVariant=InternalTs  TsampNgainVariant=Passthrough  TsampIntegralVariant=Passthrough  ExternalSaturationOutDataTypeStr=Inherit: Same as second input
  Rate Limiter : RateLimiter  SampleTimeMode=inherited
  Second-Order Filter : spsSecondOrderFilterLib/Second-Order Filter  FilterType=Lowpass  Fo=120  Zeta=0.707  Ts=Tss  Initialize=on  Vac_Init="[0,  0,  60]"  Vdc_Init=0  PlotResponse=off  FreqRange=[0, 500, 1]
      settings: SourceProductBaseCode=PS
  Sum : Sum  Inputs=|++
  abc to dq0 : spsabctodq0Lib/abc to dq0  Alignment=90 degrees behind phase A axis
  d : Outport
  q : Outport  Port=2
  f : Outport  Port=3
  wt : Outport  Port=4
  wires:
  A/1 -> Mux/1
  B/1 -> Mux/2
  C/1 -> Mux/3
  Mux/1 -> abc to dq0/1
  abc to dq0/1 -> Demux2/1
  Demux2/1 -> First-Order Filter/1, d/1
  Demux2/2 -> First-Order Filter1/1, q/1
  First-Order Filter1/1 -> Divide/2
  Divide/1 -> PID Controller1/1
  PID Controller1/1 -> Sum/1
  Second-Order Filter/1 -> Rate Limiter/1
  Normalization/1 -> Divide/1
  First-Order Filter/1 -> Normalization/1
  Sum/1 -> Discrete-Time Integrator/1, Second-Order Filter/1
  Discrete-Time Integrator/1 -> wt/1, abc to dq0/2
  Rate Limiter/1 -> f/1
  [w] -> Sum/2
  Demux2/3 -> Display/1

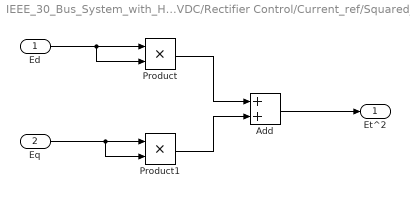
== system IEEE_30_Bus_System_with_HVDC/Rectifier Control/Current_ref/Squared_Vt ==
  Ed : Inport
  Eq : Inport  Port=2
  Add : Sum
  Product : Product
  Product1 : Product
  Et^2 : Outport
  wires:
  Ed/1 -> Product/2, Product/1
  Eq/1 -> Product1/2, Product1/1
  Add/1 -> Et^2/1
  Product/1 -> Add/1
  Product1/1 -> Add/2

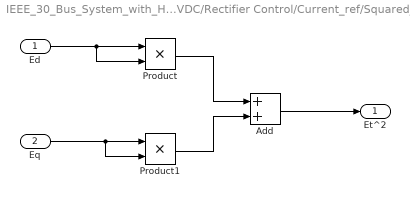
== system IEEE_30_Bus_System_with_HVDC/Rectifier Control/Current_ref/Squared_Vt1 ==
  Ed : Inport
  Eq : Inport  Port=2
  Add : Sum
  Product : Product
  Product1 : Product
  Et^2 : Outport
  wires:
  Ed/1 -> Product/2, Product/1
  Eq/1 -> Product1/2, Product1/1
  Add/1 -> Et^2/1
  Product/1 -> Add/1
  Product1/1 -> Add/2
